simulink subsystem "AccumulatorManagementRing_subsysref"  (R2020a)
settings: Solver=VariableStepAuto  StartTime=0.0  StopTime=10.0  RelTol=1e-3
undefined symbols (not defined in the file): AMR, ModelSimTime, RING_STATUS
libraries: moving_average x2, discrete_timer x2, commutil2 x1, simulink x1
settings Model: Creator=Kiera  LastModifiedBy=Kiera

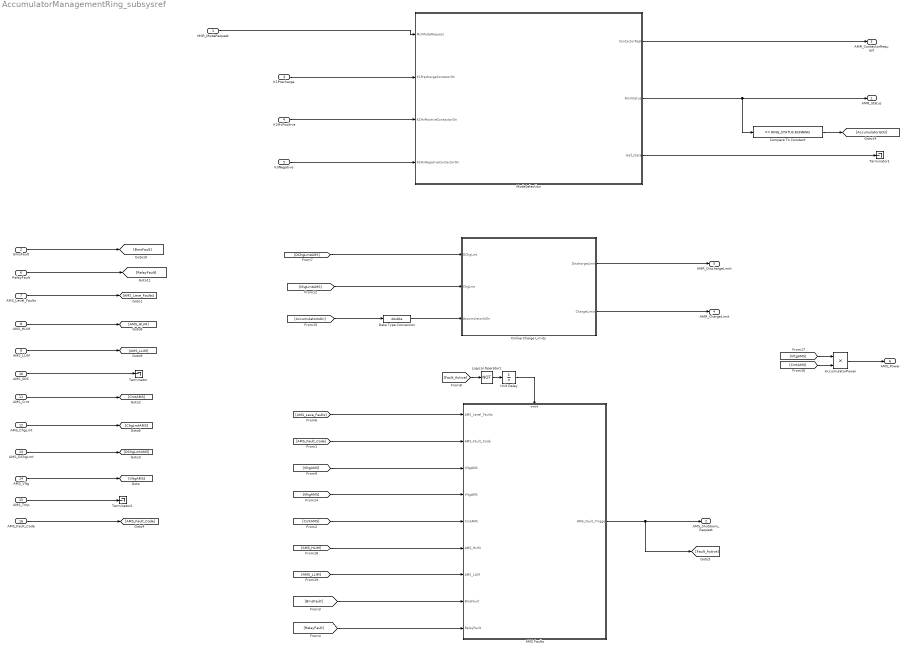
== system AccumulatorManagementRing_subsysref ==
  MSR_ModeRequest : Inport  RequirementInfo={} %GIDa_707f7e82_1f57_4317_ba83_f20165482cb4
  BmsFault : Inport  RequirementInfo={} %GIDa_99073bb8_8a3f_4198_820b_cfed4937f444  Port=2
  K1Precharge : Inport  RequirementInfo={} %GIDa_8ee29291_ac74_414d_92fe_21bcfc0c35a4  Port=3
  K2HvPositive : Inport  RequirementInfo={} %GIDa_da0d983c_f2ea_45ef_a3b7_deb856c8ae35  Port=4
  K3Negative : Inport  RequirementInfo={} %GIDa_ed5ed957_f754_4b23_bba6_8a6103de0f19  Port=5
  RelayFault : Inport  RequirementInfo={} %GIDa_ece7a76e_8156_40bc_8fe3_34ff155077e3  Port=6
  AMS_Level_Faults : Inport  RequirementInfo={} %GIDa_7ec4d0d6_7ab5_4dc4_9306_e68362cefccf  Port=7  OutDataTypeStr=uint8
  AMS_HLIM : Inport  RequirementInfo={} %GIDa_27fe7a2d_aa13_4a1d_a2c2_3f40f9dc34cc  Port=8
  AMS_LLIM : Inport  RequirementInfo={} %GIDa_1b656daa_552d_483a_8171_6e72ee90ea1d  Port=9
  AMS_SOC : Inport  RequirementInfo={} %GIDa_37fa27f2_32e3_4188_a0d8_227b6f3dd6a8  Port=10
  AMS_Crnt : Inport  RequirementInfo={} %GIDa_c46e000c_5bfa_45ad_8d8a_3ba1d49f68a6  Port=11
  AMS_ChgLmt : Inport  RequirementInfo={} %GIDa_cc1acfc0_07ee_4517_8e64_fe1326b8f01e  Port=12  OutDataTypeStr=double
  AMS_DChgLmt : Inport  RequirementInfo={} %GIDa_96ab930e_bb91_4e33_9780_3e7fc3738b34  Port=13  OutDataTypeStr=double
  AMS_Vltg : Inport  RequirementInfo={} %GIDa_2016b097_55f3_47f0_a7ad_315462987813  Port=14
  AMS_Tmp : Inport  RequirementInfo={} %GIDa_77dae94c_b313_4949_be3d_a94a36804f0e  Port=15
  AMS_Fault_Code : Inport  RequirementInfo={} %GIDa_6c4cc22a_f990_42ed_a23c_3cee6dccf86d  Port=16  OutDataTypeStr=uint8
  " ModeSelection" : Stateflow chart  RequirementInfo={} %GIDa_a096134c_4b71_44ca_8b93_4c11c62b7f49  TreatAsAtomicUnit=on
  AMS Faults : Subsystem  RequirementInfo={} %GIDa_d4f403b1_51e7_4ccc_bdca_545d4acd8941
  AccumulatorPower : Product  RequirementInfo={} %GIDa_e046f157_11bf_4661_9472_3b0a4da84df8
  Compare To Constant : simulink/Logic and Bit Operations/Compare To Constant  relop===  const=RING_STATUS.RUNNING  OutDataTypeStr=boolean
  Data Type Conversion : DataTypeConversion  RequirementInfo={} %GIDa_8ceb1c07_8cfc_4b92_8da2_d1080dfa1b56  OutDataTypeStr=double
  Logical Operator1 : Logic  RequirementInfo={} %GIDa_05af19c6_7032_4869_992b_9d906616b0d9  Operator=NOT  AllPortsSameDT=off  OutDataTypeStr=boolean
  Online Charge Limits : Subsystem  RequirementInfo={'linktype_rmi_slreq' 'AmrRequirements.slreqx' '3' 'true' 'Checks Voltage (AmrRequirements#3)' '' } %GIDa_b8824ce6_1bf8_4ced_8633_7304403eefc3
  Terminator : Terminator
      settings: RequirementInfo={} %GIDa_b0f769aa_c909_43b3_ae21_8f787d138f48
  Terminator1 : Terminator
      settings: RequirementInfo={} %GIDa_0f881a05_a580_4d46_9939_f06e6a6f1128
  Terminator2 : Terminator
      settings: RequirementInfo={} %GIDa_47c18584_9fb7_46d4_b73f_bd4de39157eb
  Unit Delay : UnitDelay  RequirementInfo={} %GIDa_2608e194_dac7_44b8_8e49_fc2e06511837  SampleTime=-1  HasFrameUpgradeWarning=on
  AMR_Status : Outport  RequirementInfo={} %GIDa_8de4b995_749e_4c4c_afbc_3fa3bf134919  VectorParamsAs1DForOutWhenUnconnected=off
  AMS_Shutdown_Request : Outport  RequirementInfo={} %GIDa_0ae9fa20_6cc3_411d_ba6b_023417513ac9  Port=2  VectorParamsAs1DForOutWhenUnconnected=off
  AMR_ContactorRequest : Outport  RequirementInfo={} %GIDa_2e1744d9_8f28_4491_9f6a_543804bfa97a  Port=3  VectorParamsAs1DForOutWhenUnconnected=off
  AMR_ChargeLimit : Outport  RequirementInfo={} %GIDa_b6207ed3_6282_4168_b685_e6f38b5ce99f  Port=4  VectorParamsAs1DForOutWhenUnconnected=off
  AMR_DischargeLimit : Outport  RequirementInfo={} %GIDa_6aff832c_991b_419e_a563_e35d0ab09dd6  Port=5  VectorParamsAs1DForOutWhenUnconnected=off
  AMS_Power : Outport  RequirementInfo={} %GIDa_5c1d55a2_9c3b_4dcb_ab01_704b593d1249  Port=6  VectorParamsAs1DForOutWhenUnconnected=off
  wires:
  Unit Delay/1 -> AMS Faults/Enable
  K2HvPositive/1 -> " ModeSelection"/3(K2HvPositiveContactorOn)
  AMS_ChgLmt/1 -> [ChgLmtAMS]
  K1Precharge/1 -> " ModeSelection"/2(K1PrechargeContatorOn)
  [CrntAMS] -> AMS Faults/5(CrntAMS)
  [AMS_Leve_Faults] -> AMS Faults/1(AMS_Level_Faults)
  Logical Operator1/1 -> Unit Delay/1
  [RelayFault] -> AMS Faults/9(RelayFault)
  AMS Faults/1("AMS_Fault_Trigger ") -> AMS_Shutdown_Request/1, [Fault_Active]
  [BmsFault] -> AMS Faults/8(BmsFault)
  RelayFault/1 -> [RelayFault]
  [AMS_Fault_Code] -> AMS Faults/2(AMS_Fault_Code)
  BmsFault/1 -> [BmsFault]
  Data Type Conversion/1 -> Online Charge Limits/3(AccumulatorIsOn)
  [VltgAMS] -> AMS Faults/4(VltgAMS)
  Compare To Constant/1 -> [AccumulatorIsOn]
  [Fault_Active] -> Logical Operator1/1
  AccumulatorPower/1 -> AMS_Power/1
  AMS_Vltg/1 -> [VltgAMS]
  AMS_SOC/1 -> Terminator/1
  MSR_ModeRequest/1 -> " ModeSelection"/1(MsrModeRequest)
  " ModeSelection"/3(leaf_state) -> Terminator1/1
  Online Charge Limits/2(ChargeLimit) -> AMR_ChargeLimit/1
  [AMS_HLIM] -> AMS Faults/6(AMS_HLIM)
  [ChgLmtAMS] -> Online Charge Limits/2(ChgLmt)
  [DChgLmtAMS] -> Online Charge Limits/1(DChgLmt)
  AMS_LLIM/1 -> [AMS_LLIM]
  [VltgAMS] -> AMS Faults/3("VltgAMS ")
  [AccumulatorIsOn] -> Data Type Conversion/1
  " ModeSelection"/2(AmrStatus) -> Compare To Constant/1, AMR_Status/1
  AMS_Fault_Code/1 -> [AMS_Fault_Code]
  AMS_DChgLmt/1 -> [DChgLmtAMS]
  [AMS_LLIM] -> AMS Faults/7(AMS_LLIM)
  AMS_Tmp/1 -> Terminator2/1
  Online Charge Limits/1(DischargeLimit) -> AMR_DischargeLimit/1
  " ModeSelection"/1(ContactorRqst) -> AMR_ContactorRequest/1
  AMS_Level_Faults/1 -> [AMS_Leve_Faults]
  AMS_Crnt/1 -> [CrntAMS]
  [VltgAMS] -> AccumulatorPower/1
  K3Negative/1 -> " ModeSelection"/4(K3HvNegativeContactorOn)
  [CrntAMS] -> AccumulatorPower/2
  AMS_HLIM/1 -> [AMS_HLIM]

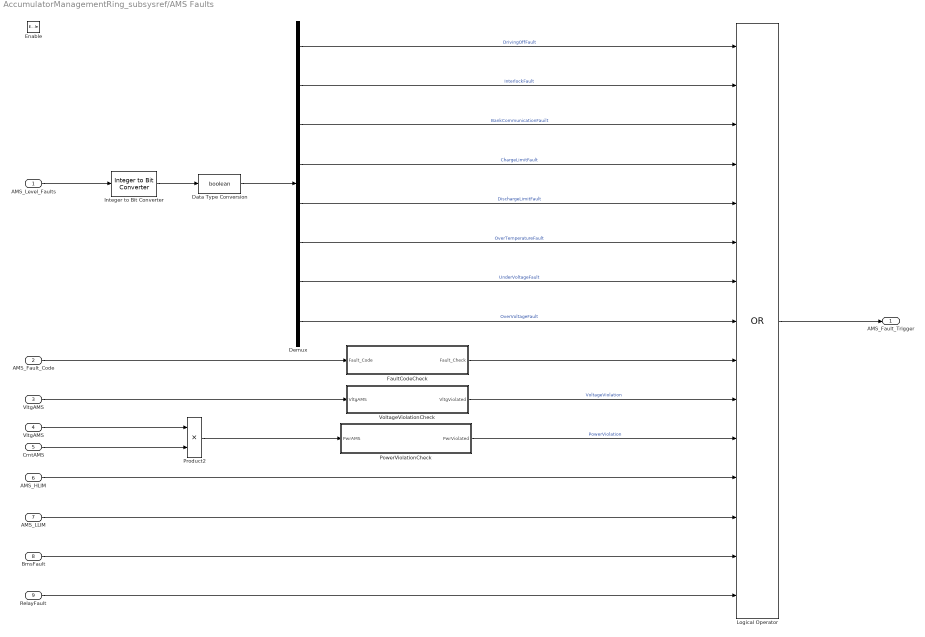
== system AccumulatorManagementRing_subsysref/AMS Faults ==
  AMS_Level_Faults : Inport  RequirementInfo={} %GIDa_e0aa747c_ba5b_40eb_b723_0b9efbfcd836
  AMS_Fault_Code : Inport  RequirementInfo={} %GIDa_0ce65da5_0176_4ad7_9433_4bafd1cb0cc0  Port=2
  "VltgAMS " : Inport  RequirementInfo={} %GIDa_16765c4f_aed4_4f03_8ea8_e83820a37110  Port=3
  VltgAMS : Inport  RequirementInfo={} %GIDa_2ff50595_b0bb_403d_9a6f_26094e66622e  Port=4
  CrntAMS : Inport  RequirementInfo={} %GIDa_b2853c49_3d6b_4e00_935d_399f01de6206  Port=5
  AMS_HLIM : Inport  RequirementInfo={} %GIDa_57aba87d_602d_415f_9ccf_9082aa6107e6  Port=6
  AMS_LLIM : Inport  RequirementInfo={} %GIDa_711fc5be_7daf_4273_b649_f557f235f411  Port=7
  BmsFault : Inport  RequirementInfo={} %GIDa_9d859fbf_f12d_4c50_9b90_e59e5f90d7f1  Port=8
  RelayFault : Inport  RequirementInfo={} %GIDa_41ac8945_f063_4f40_90f4_7400c54ef034  Port=9
  Enable : EnablePort  RequirementInfo={} %GIDa_97d485e2_6103_4895_b31c_550f181b7117
  Data Type Conversion : DataTypeConversion  RequirementInfo={} %GIDa_5c9141ea_0ff7_49ad_bba4_f9bfb3a7a1e2  OutDataTypeStr=boolean
  Demux : Demux  RequirementInfo={} %GIDa_221c6b5a_cf4a_4757_bb19_40a7011ba5d5  Outputs=8
  FaultCodeCheck : Subsystem  RequirementInfo={} %GIDa_864cb63c_e5e9_4231_b8d7_1003b5a76e85
  Integer to Bit Converter : commutil2/Integer to Bit Converter  RequirementInfo={} %GIDa_7c43af0b_e99f_4b9e_99bd_f0926f09c729  nbits=8  signedInputValues=Unsigned  bitOrder=LSB first  outDtype=Inherit via internal rule
  Logical Operator : Logic  RequirementInfo={} %GIDa_17e4bb28_e737_45cb_8170_889f61b36965  Operator=OR  Inputs=15  AllPortsSameDT=off  OutDataTypeStr=boolean
  "PowerViolationCheck " : Subsystem  RequirementInfo={} %GIDa_abf1642e_4fd0_4974_b913_3294f86b6ad1
  Product2 : Product  RequirementInfo={} %GIDa_4829654b_2af4_48c3_8d35_7114d49d1942
  VoltageViolationCheck : Subsystem  RequirementInfo={} %GIDa_caa66ec5_5711_49d5_b1f9_896aea5d9348
  "AMS_Fault_Trigger " : Outport  RequirementInfo={} %GIDa_38164578_59d1_49cd_8022_3d2d3f1a8b39  VectorParamsAs1DForOutWhenUnconnected=off
  wires:
  Integer to Bit Converter/1 -> Data Type Conversion/1
  AMS_Level_Faults/1 -> Integer to Bit Converter/1
  Data Type Conversion/1 -> Demux/1
  AMS_Fault_Code/1 -> FaultCodeCheck/1(Fault_Code)
  Product2/1 -> "PowerViolationCheck "/1(PwrAMS)
  VltgAMS/1 -> Product2/1
  "VltgAMS "/1 -> VoltageViolationCheck/1(VltgAMS)
  CrntAMS/1 -> Product2/2
  Demux/1 -> Logical Operator/1  "DrivingOffFault"
  Demux/2 -> Logical Operator/2  "InterlockFault"
  Demux/3 -> Logical Operator/3  "BankCommunicationFauilt"
  Demux/4 -> Logical Operator/4  "ChargeLimitFault"
  Demux/5 -> Logical Operator/5  "DischargeLimitFault"
  Demux/6 -> Logical Operator/6  "OverTemperatureFault"
  Demux/7 -> Logical Operator/7  "UnderVoltageFault"
  Demux/8 -> Logical Operator/8  "OverVoltageFault"
  FaultCodeCheck/1(Fault_Check) -> Logical Operator/9
  VoltageViolationCheck/1(VltgViolated) -> Logical Operator/10  "VoltageViolation"
  "PowerViolationCheck "/1(PwrViolated) -> Logical Operator/11  "PowerViolation"
  Logical Operator/1 -> "AMS_Fault_Trigger "/1
  AMS_HLIM/1 -> Logical Operator/12
  AMS_LLIM/1 -> Logical Operator/13
  BmsFault/1 -> Logical Operator/14
  RelayFault/1 -> Logical Operator/15

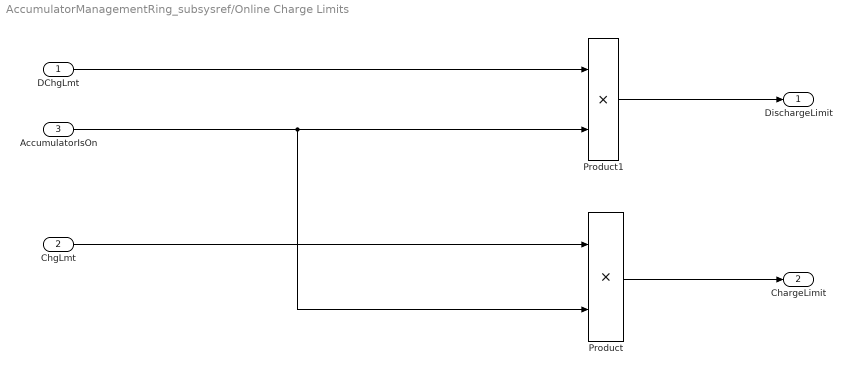
== system AccumulatorManagementRing_subsysref/Online Charge Limits ==
  DChgLmt : Inport  RequirementInfo={} %GIDa_365715b9_38a1_4f91_99b2_dba1e028ba9d
  ChgLmt : Inport  RequirementInfo={} %GIDa_4459bc43_4753_44df_a821_233b41f898ac  Port=2
  AccumulatorIsOn : Inport  RequirementInfo={} %GIDa_5f533cce_dc63_4241_a88f_dcb6e64eec05  Port=3
  Product : Product  RequirementInfo={} %GIDa_dd5b4ffe_4cc2_4dc7_97fb_fb0363f245db
  Product1 : Product  RequirementInfo={} %GIDa_a2aaec0c_b480_4bee_a4ba_58ab46f570bf
  DischargeLimit : Outport  RequirementInfo={} %GIDa_bab987c6_0aa0_4acd_992d_1be6464b7e53  VectorParamsAs1DForOutWhenUnconnected=off
  ChargeLimit : Outport  RequirementInfo={} %GIDa_1f63c40f_9b8f_4f81_9e04_f3fa4adf6511  Port=2  VectorParamsAs1DForOutWhenUnconnected=off
  wires:
  AccumulatorIsOn/1 -> Product/2, Product1/2
  ChgLmt/1 -> Product/1
  Product/1 -> ChargeLimit/1
  DChgLmt/1 -> Product1/1
  Product1/1 -> DischargeLimit/1

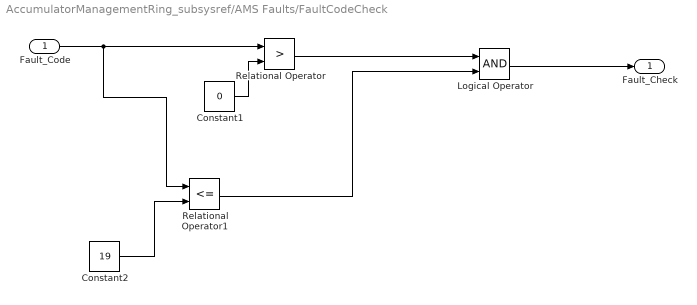
== system AccumulatorManagementRing_subsysref/AMS Faults/FaultCodeCheck ==
  Fault_Code : Inport  RequirementInfo={} %GIDa_08cc9594_68f8_46b6_ae36_619b9983c707
  Constant1 : Constant  RequirementInfo={} %GIDa_44fedb71_3525_4aa7_a046_07e76cab7cf7  Value=0
  Constant2 : Constant  RequirementInfo={} %GIDa_ecb20799_8931_46d6_9b6d_78defff3dc69  Value=19
  Logical Operator : Logic  RequirementInfo={} %GIDa_974e838d_edcc_428d_af46_c097c4445dfb  AllPortsSameDT=off  OutDataTypeStr=boolean
  Relational Operator : RelationalOperator  RequirementInfo={} %GIDa_fc61807c_a972_402d_a1fc_7824d6d4bc63  Operator=>  OutDataTypeStr=boolean  RndMeth=Simplest
  Relational Operator1 : RelationalOperator  RequirementInfo={} %GIDa_436b65fa_949c_4445_b41b_812697c81fd2  Operator=<=  OutDataTypeStr=boolean  RndMeth=Simplest
  Fault_Check : Outport  RequirementInfo={} %GIDa_616f0ff8_0eda_4bb9_843f_7d99ce111c24  VectorParamsAs1DForOutWhenUnconnected=off
  wires:
  Fault_Code/1 -> Relational Operator1/1, Relational Operator/1
  Constant1/1 -> Relational Operator/2
  Constant2/1 -> Relational Operator1/2
  Relational Operator1/1 -> Logical Operator/2
  Relational Operator/1 -> Logical Operator/1
  Logical Operator/1 -> Fault_Check/1

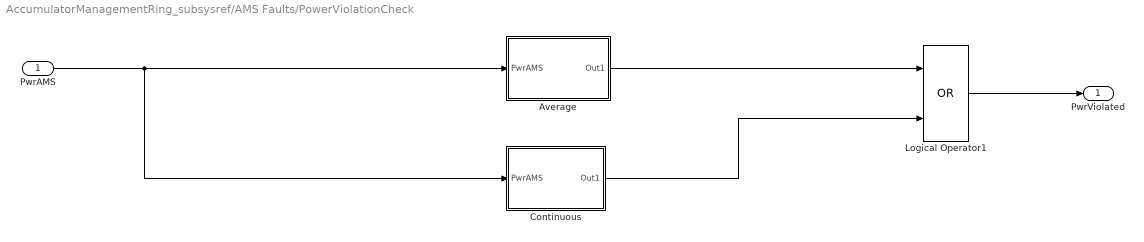
== system AccumulatorManagementRing_subsysref/AMS Faults/PowerViolationCheck  ==
  PwrAMS : Inport  RequirementInfo={} %GIDa_8482f58d_d744_4ae9_81f4_668f1214485b
  Average : Subsystem  RequirementInfo={} %GIDa_a259fab0_46bc_4c1a_8bcd_31dd5d9bfba1
  Continuous : Subsystem  RequirementInfo={} %GIDa_afab7bfa_631b_4528_8dd3_c32b116153f0
  Logical Operator1 : Logic  RequirementInfo={} %GIDa_8e4819b7_6247_4944_8665_944a6715c190  Operator=OR  AllPortsSameDT=off  OutDataTypeStr=boolean
  PwrViolated : Outport  RequirementInfo={} %GIDa_11f78fc0_f29f_4b9a_9cdd_9632dc7ef126  VectorParamsAs1DForOutWhenUnconnected=off
  wires:
  Logical Operator1/1 -> PwrViolated/1
  PwrAMS/1 -> Continuous/1(PwrAMS), Average/1(PwrAMS)
  Average/1(Out1) -> Logical Operator1/1
  Continuous/1(Out1) -> Logical Operator1/2

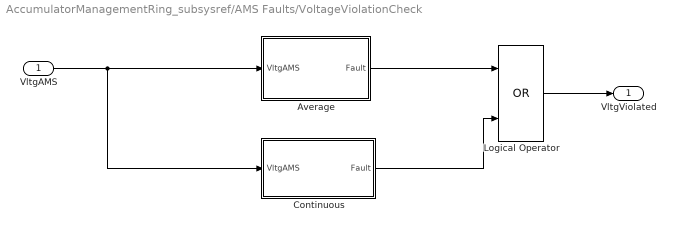
== system AccumulatorManagementRing_subsysref/AMS Faults/VoltageViolationCheck ==
  VltgAMS : Inport  RequirementInfo={} %GIDa_6396be71_42a8_41f8_b8a7_9994d47d1ca1
  Average : Subsystem  RequirementInfo={} %GIDa_8ad955fb_06fc_49d9_ba91_c2127422c577
  Continuous : Subsystem  RequirementInfo={} %GIDa_f5a5810f_ed1e_496b_96b3_a189fc7dd252
  Logical Operator : Logic  RequirementInfo={} %GIDa_ae595f51_bfc1_48b2_a9f1_ac933bd19462  Operator=OR  AllPortsSameDT=off  OutDataTypeStr=boolean
  VltgViolated : Outport  RequirementInfo={} %GIDa_e19ac1ad_ed7a_4695_bb68_aadc67f16c69  VectorParamsAs1DForOutWhenUnconnected=off
  wires:
  Logical Operator/1 -> VltgViolated/1
  Average/1(Fault) -> Logical Operator/1
  Continuous/1(Fault) -> Logical Operator/2
  VltgAMS/1 -> Continuous/1(VltgAMS), Average/1(VltgAMS)

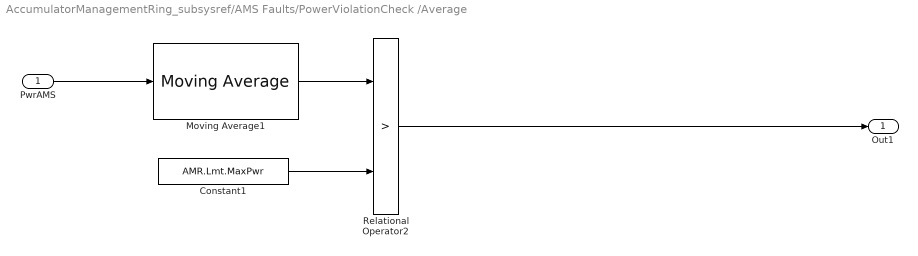
== system AccumulatorManagementRing_subsysref/AMS Faults/PowerViolationCheck /Average ==
  PwrAMS : Inport  RequirementInfo={} %GIDa_85e9fc51_b6fc_4c14_a950_dfd6c32c835c
  Constant1 : Constant  RequirementInfo={} %GIDa_4c495632_9687_47ef_b02c_c930a0dbe2f4  Value=AMR.Lmt.MaxPwr
  Moving Average1 : moving_average/Moving Average  SampleTime=ModelSimTime  WindowSize=AMR.Lmt.Tavg
  Relational Operator2 : RelationalOperator  RequirementInfo={} %GIDa_b79d5c37_d4b6_42dd_a6f1_c420555bb0c0  Operator=>  OutDataTypeStr=boolean  RndMeth=Nearest
  Out1 : Outport  RequirementInfo={} %GIDa_6e7a77de_09b0_4030_85ce_7bd50d1fc273  VectorParamsAs1DForOutWhenUnconnected=off
  wires:
  Relational Operator2/1 -> Out1/1
  Constant1/1 -> Relational Operator2/2
  Moving Average1/1 -> Relational Operator2/1
  PwrAMS/1 -> Moving Average1/1

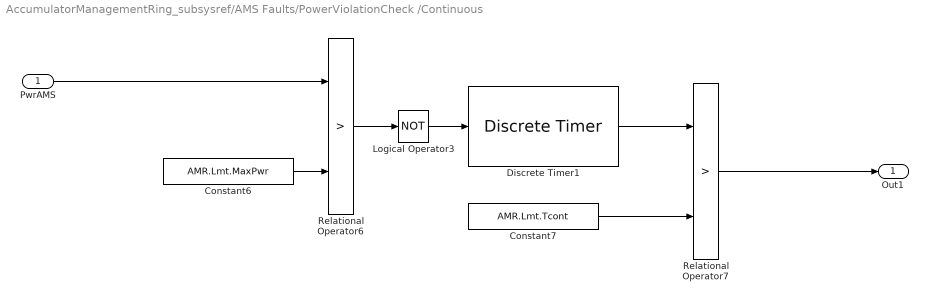
== system AccumulatorManagementRing_subsysref/AMS Faults/PowerViolationCheck /Continuous ==
  PwrAMS : Inport  RequirementInfo={} %GIDa_860820aa_8b20_48b4_99b3_bc30178b06fd
  Constant6 : Constant  RequirementInfo={} %GIDa_5702958b_0bfa_4962_98db_bdeedc8fd614  Value=AMR.Lmt.MaxPwr
  Constant7 : Constant  RequirementInfo={} %GIDa_694739ad_8ee1_401f_9c05_c4d2506a53a8  Value=AMR.Lmt.Tcont
  Discrete Timer1 : discrete_timer/Discrete Timer  RequirementInfo={} %GIDa_c12e57c1_81b8_4b5c_922b_f4e616a676f8
  Logical Operator3 : Logic  RequirementInfo={} %GIDa_61cb6828_0bfb_4203_add9_67042e976126  Operator=NOT  AllPortsSameDT=off  OutDataTypeStr=boolean
  Relational Operator6 : RelationalOperator  RequirementInfo={} %GIDa_311dd147_4fa1_4e34_9c9e_14ab067d7b2d  Operator=>  OutDataTypeStr=boolean  RndMeth=Nearest
  Relational Operator7 : RelationalOperator  RequirementInfo={} %GIDa_3f612e11_950e_4ea6_8537_cd02068fdbe1  Operator=>  OutDataTypeStr=boolean  RndMeth=Nearest
  Out1 : Outport  RequirementInfo={} %GIDa_3d537400_c7c0_4702_9562_89720a581e51  VectorParamsAs1DForOutWhenUnconnected=off
  wires:
  Logical Operator3/1 -> Discrete Timer1/1
  Relational Operator7/1 -> Out1/1
  Relational Operator6/1 -> Logical Operator3/1
  Constant6/1 -> Relational Operator6/2
  Discrete Timer1/1 -> Relational Operator7/1
  Constant7/1 -> Relational Operator7/2
  PwrAMS/1 -> Relational Operator6/1

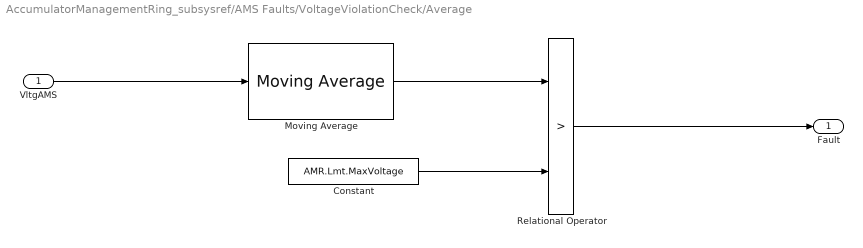
== system AccumulatorManagementRing_subsysref/AMS Faults/VoltageViolationCheck/Average ==
  VltgAMS : Inport  RequirementInfo={} %GIDa_8d7cacfc_f285_43d6_a10e_496117ec5010
  Constant : Constant  RequirementInfo={} %GIDa_140e8be5_fd1d_4bc0_9fcf_140c440f9cab  Value=AMR.Lmt.MaxVoltage
  Moving Average : moving_average/Moving Average  SampleTime=ModelSimTime  WindowSize=AMR.Lmt.Tavg
  Relational Operator : RelationalOperator  RequirementInfo={} %GIDa_55512027_80d1_47cc_9232_3c254380ffa8  Operator=>  OutDataTypeStr=boolean  RndMeth=Nearest
  Fault : Outport  RequirementInfo={} %GIDa_61a96bfd_3017_41e8_b46a_97f30d9d01ef  VectorParamsAs1DForOutWhenUnconnected=off
  wires:
  Moving Average/1 -> Relational Operator/1
  VltgAMS/1 -> Moving Average/1
  Constant/1 -> Relational Operator/2
  Relational Operator/1 -> Fault/1

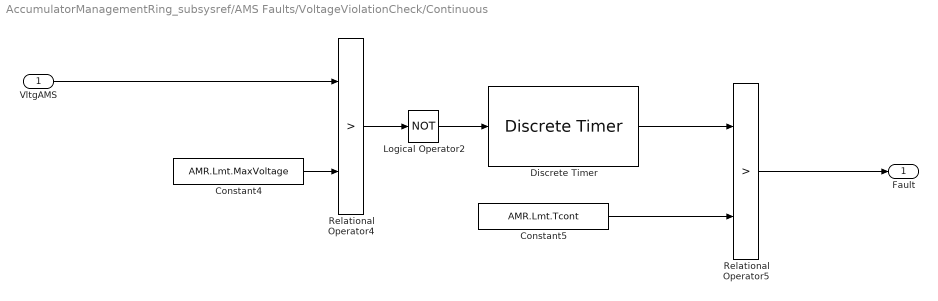
== system AccumulatorManagementRing_subsysref/AMS Faults/VoltageViolationCheck/Continuous ==
  VltgAMS : Inport  RequirementInfo={} %GIDa_d844e947_8e58_46cb_b895_70c0a2d5ca5b
  Constant4 : Constant  RequirementInfo={} %GIDa_b42a1fe5_1ead_40ff_bab2_02ff39506114  Value=AMR.Lmt.MaxVoltage
  Constant5 : Constant  RequirementInfo={} %GIDa_efccf25d_5577_45f5_9eed_34127ebced7f  Value=AMR.Lmt.Tcont
  Discrete Timer : discrete_timer/Discrete Timer
  Logical Operator2 : Logic  RequirementInfo={} %GIDa_f6ebf125_f3da_43ae_ae3c_65018c5708ab  Operator=NOT  AllPortsSameDT=off  OutDataTypeStr=boolean
  Relational Operator4 : RelationalOperator  RequirementInfo={} %GIDa_bae890ad_1273_40e3_a2f4_f7b6b4832ff2  Operator=>  OutDataTypeStr=boolean  RndMeth=Nearest
  Relational Operator5 : RelationalOperator  RequirementInfo={} %GIDa_52e5f431_970f_43b5_9f9c_9ab6f1c43f28  Operator=>  OutDataTypeStr=boolean  RndMeth=Nearest
  Fault : Outport  RequirementInfo={} %GIDa_fe5f5458_4915_4647_b043_7781a6e3f041  VectorParamsAs1DForOutWhenUnconnected=off
  wires:
  Logical Operator2/1 -> Discrete Timer/1
  Relational Operator4/1 -> Logical Operator2/1
  Relational Operator5/1 -> Fault/1
  Constant5/1 -> Relational Operator5/2
  Discrete Timer/1 -> Relational Operator5/1
  Constant4/1 -> Relational Operator4/2
  VltgAMS/1 -> Relational Operator4/1

== stateflow chart AccumulatorManagementRing_subsysref/ ModeSelection ==
  state Shutdown
    en:
    state ShutdownInProgress
      entry:
      AmrStatus = RING_STATUS.SHUTDOWN_IN_PROGRESS_HV;
      ContactorRqst = 0;
    state ShutdownComplete
      entry:
      AmrStatus = RING_STATUS.SHUTDOWN_COMPLETE_HV;
    (default) -> ShutdownInProgress
    ShutdownInProgress -> ShutdownComplete : [~K1PrechargeContatorOn &&...
        | ~K2HvPositiveContactorOn &&...
        | ~K3HvNegativeContactorOn]
  state Off
    entry:
    ContactorRqst = 0;
    AmrStatus = RING_STATUS.OFF;
  state OPERATIONAL
    state Startup
      state RqstPrechg
        entry:
        AmrStatus = RING_STATUS.STARTUP_IN_PROGRESS_HV;
        ContactorRqst = 1;
      state HVPrechg
        entry:
      state HVComplete
        entry:
        AmrStatus = RING_STATUS.STARTUP_COMPLETE_HV;
      (default) -> RqstPrechg
      RqstPrechg -> HVPrechg : [K1PrechargeContatorOn &&...
          | ~K2HvPositiveContactorOn &&...
          | K3HvNegativeContactorOn]
      HVPrechg -> HVComplete : [~K1PrechargeContatorOn &&...
          | K2HvPositiveContactorOn &&...
          | K3HvNegativeContactorOn]
    state Running
      entry:
      AmrStatus = RING_STATUS.RUNNING;
      % No checks are implemented to keep the system as simple as possible
    (default) -> Startup
    Startup -> Running : [MsrModeRequest == MSR_REQUEST.RUNNING && AmrStatus == RING_STATUS.STARTUP_COMPLETE_HV]
  (default) -> Off
  Off -> OPERATIONAL : [MsrModeRequest == MSR_REQUEST.STARTUP_HV]
  OPERATIONAL -> Shutdown : [MsrModeRequest == MSR_REQUEST.SHUTDOWN_HV]
  data: MsrModeRequest input Enum: MSR_REQUEST; ContactorRqst output; K1PrechargeContatorOn input boolean; AmrStatus output Enum: RING_STATUS; leaf_state output Enum: AMR_leaf_states; K2HvPositiveContactorOn input boolean; K3HvNegativeContactorOn input boolean
